simulink model "NegativeSpringSim_R2017a"  (R2017a)
settings: Solver=FixedStepAuto  StartTime=0.0  StopTime=10.0  FixedStep=Ts  RelTol=1e-3
undefined symbols (not defined in the file): Ha, k, Kd, Ki, Kp, m, N
libraries: simulink x1, cstblocks x1
settings Model: Creator=XiaoCY  LastModifiedBy=XiaoCY
settings SFSimCC: SimUseLocalCustomCode=on
settings RTWCC: RTWUseLocalCustomCode=on

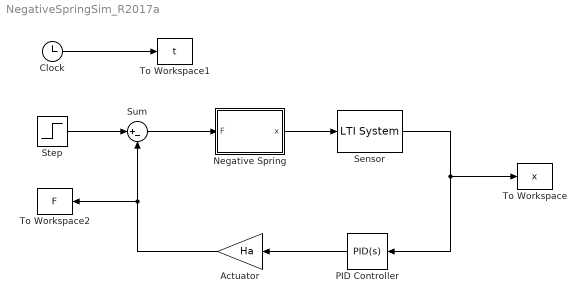
== system NegativeSpringSim_R2017a ==
  Actuator : Gain  Gain=Ha
  Clock : Clock
  Negative Spring : Subsystem
  PID Controller : simulink/Continuous/PID Controller  Controller=PID  Form=Ideal  TimeDomain=Continuous-time  SampleTime=-1  IntegratorMethod=Forward Euler  FilterMethod=Forward Euler  ControllerParametersSource=internal  P=Kp  I=Ki  D=Kd  UseFilter=on  N=N  InitialConditionSource=internal  InitialConditionForIntegrator=0  InitialConditionForFilter=0  DifferentiatorICPrevScaledInput=0  ExternalReset=none  TrackingMode=off  Kt=1  LimitOutput=off  UpperSaturationLimit=inf  LowerSaturationLimit=-inf  LinearizeAsGain=on  AntiWindupMode=none  Kb=1  POutMin=[]  POutMax=[]  IOutMin=[]  IOutMax=[]  DOutMin=[]  DOutMax=[]  NOutMin=[]  NOutMax=[]  SumOutMin=[]  SumOutMax=[]  SaturationOutMin=[]  SaturationOutMax=[]  PParamMin=[]  PParamMax=[]  IParamMin=[]  IParamMax=[]  DParamMin=[]  DParamMax=[]  NParamMin=[]  NParamMax=[]  KbParamMin=[]  KbParamMax=[]  KtParamMin=[]  KtParamMax=[]  KbOutMin=[]  KbOutMax=[]  KtOutMin=[]  KtOutMax=[]  IntegratorOutMin=[]  IntegratorOutMax=[]  FilterOutMin=[]  FilterOutMax=[]  SumI1OutMin=[]  SumI1OutMax=[]  SumI2OutMin=[]  SumI2OutMax=[]  SumI3OutMin=[]  SumI3OutMax=[]  SumDOutMin=[]  SumDOutMax=[]  DifferentiatorOutMin=[]  DifferentiatorOutMax=[]  IntegratorContinuousStateAttributes=''  IntegratorStateMustResolveToSignalObject=off  IntegratorRTWStateStorageClass=Auto  FilterContinuousStateAttributes=''  FilterStateMustResolveToSignalObject=off  FilterRTWStateStorageClass=Auto
  Sensor : cstblocks/LTI System  sys=Hs  IC=[]
  Step : Step  Time=0  SampleTime=0
  Sum : Sum  Inputs=|+-
  To Workspace : ToWorkspace  VariableName=x  SampleTime=-1
  To Workspace1 : ToWorkspace  VariableName=t  SampleTime=-1
  To Workspace2 : ToWorkspace  VariableName=F  SampleTime=-1
  wires:
  Step/1 -> Sum/1
  Sum/1 -> Negative Spring/1(F)
  Negative Spring/1(x) -> Sensor/1
  Sensor/1 -> PID Controller/1, To Workspace/1
  PID Controller/1 -> Actuator/1
  Actuator/1 -> To Workspace2/1, Sum/2
  Clock/1 -> To Workspace1/1

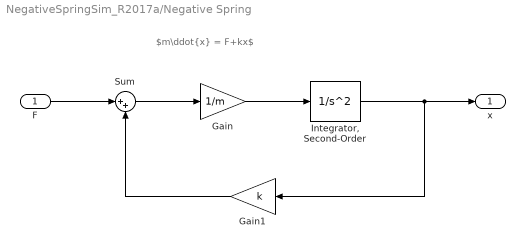
== system NegativeSpringSim_R2017a/Negative Spring ==
  note: $m\ddot{x} = F+kx$
  F : Inport
  Gain : Gain  Gain=1/m
  Gain1 : Gain  Gain=k
  "Integrator, Second-Order" : SecondOrderIntegrator  ShowOutput=x
  Sum : Sum  Inputs=|++
  x : Outport
  wires:
  F/1 -> Sum/1
  Sum/1 -> Gain/1
  Gain/1 -> "Integrator, Second-Order"/1
  "Integrator, Second-Order"/1 -> Gain1/1, x/1
  Gain1/1 -> Sum/2
